simulink library "Lib_Sensors"  (R2014b)
settings: Solver=ode45  StartTime=0.0  StopTime=10.0  RelTol=1e-3
settings Model: Creator=Ehang  LastModifiedBy=Ehang

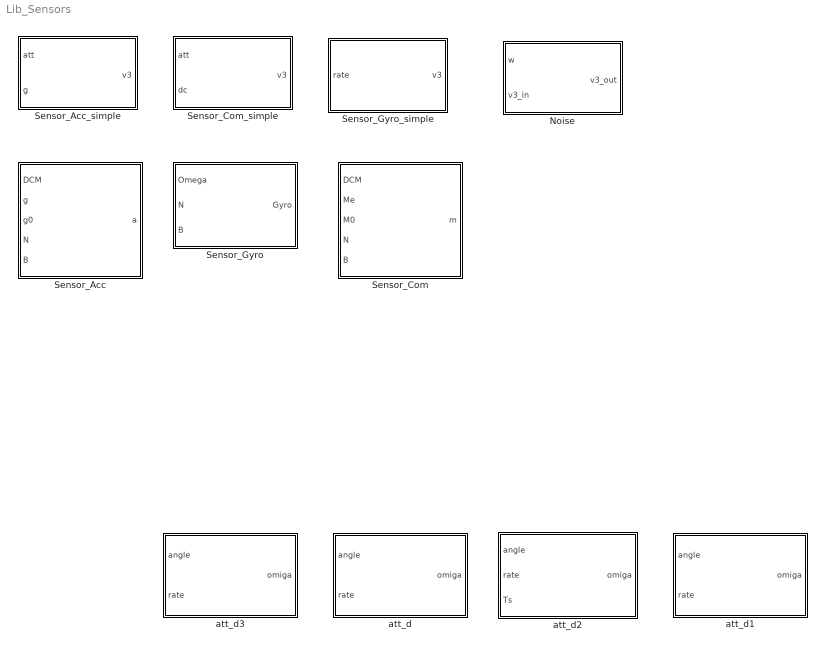
== system Lib_Sensors ==
  Noise : MATLAB Function  TreatAsAtomicUnit=on
  Sensor_Acc : Subsystem
  Sensor_Acc_simple : MATLAB Function  TreatAsAtomicUnit=on
  Sensor_Com : Subsystem
  Sensor_Com_simple : MATLAB Function  TreatAsAtomicUnit=on
  Sensor_Gyro : Subsystem
  Sensor_Gyro_simple : MATLAB Function  TreatAsAtomicUnit=on
  att_d : MATLAB Function  TreatAsAtomicUnit=on
  att_d1 : MATLAB Function  TreatAsAtomicUnit=on
  att_d2 : MATLAB Function  TreatAsAtomicUnit=on
  att_d3 : MATLAB Function  TreatAsAtomicUnit=on

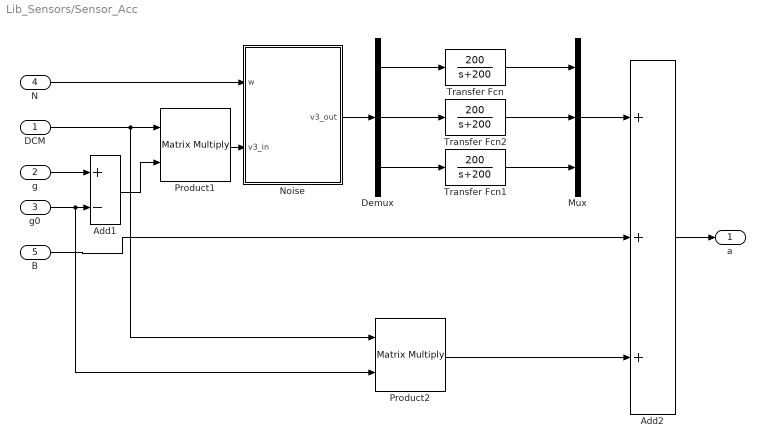
== system Lib_Sensors/Sensor_Acc ==
  DCM : Inport  PortDimensions=[3,3]
  g : Inport  Port=2
  g0 : Inport  Port=3
  N : Inport  Port=4  PortDimensions=[3,3]
  B : Inport  Port=5
  Add1 : Sum  Inputs=+-
  Add2 : Sum  Inputs=+++
  Demux : Demux  Outputs=3
  Mux : Mux  Inputs=3
  Noise : MATLAB Function  TreatAsAtomicUnit=on
  Product1 : Product  Multiplication=Matrix(*)
  Product2 : Product  Multiplication=Matrix(*)
  Transfer Fcn : TransferFcn  Numerator=[200]  Denominator=[1 200]
  Transfer Fcn1 : TransferFcn  Numerator=[200]  Denominator=[1 200]
  Transfer Fcn2 : TransferFcn  Numerator=[200]  Denominator=[1 200]
  a : Outport  PortDimensions=[3,1]
  wires:
  DCM/1 -> Product2/1, Product1/1
  Product1/1 -> Noise/2(v3_in)
  N/1 -> Noise/1(w)
  Noise/1(v3_out) -> Demux/1
  B/1 -> Add2/2
  Mux/1 -> Add2/1
  Transfer Fcn/1 -> Mux/1
  Demux/1 -> Transfer Fcn/1
  Transfer Fcn2/1 -> Mux/2
  Transfer Fcn1/1 -> Mux/3
  Demux/3 -> Transfer Fcn1/1
  Demux/2 -> Transfer Fcn2/1
  Add2/1 -> a/1
  g0/1 -> Product2/2, Add1/2
  g/1 -> Add1/1
  Add1/1 -> Product1/2
  Product2/1 -> Add2/3

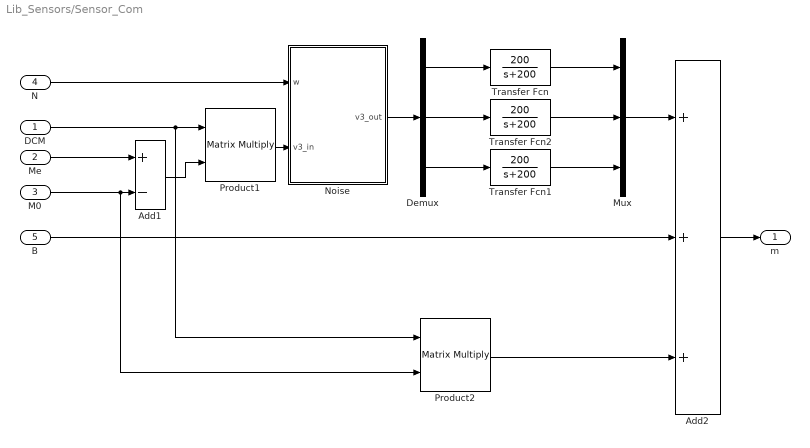
== system Lib_Sensors/Sensor_Com ==
  DCM : Inport  PortDimensions=[3,3]
  Me : Inport  Port=2
  M0 : Inport  Port=3
  N : Inport  Port=4  PortDimensions=[3,3]
  B : Inport  Port=5
  Add1 : Sum  Inputs=+-
  Add2 : Sum  Inputs=+++
  Demux : Demux  Outputs=3
  Mux : Mux  Inputs=3
  Noise : MATLAB Function  TreatAsAtomicUnit=on
  Product1 : Product  Multiplication=Matrix(*)
  Product2 : Product  Multiplication=Matrix(*)
  Transfer Fcn : TransferFcn  Numerator=[200]  Denominator=[1 200]
  Transfer Fcn1 : TransferFcn  Numerator=[200]  Denominator=[1 200]
  Transfer Fcn2 : TransferFcn  Numerator=[200]  Denominator=[1 200]
  m : Outport  PortDimensions=[3,1]
  wires:
  DCM/1 -> Product2/1, Product1/1
  Product1/1 -> Noise/2(v3_in)
  N/1 -> Noise/1(w)
  Noise/1(v3_out) -> Demux/1
  B/1 -> Add2/2
  Mux/1 -> Add2/1
  Transfer Fcn/1 -> Mux/1
  Demux/1 -> Transfer Fcn/1
  Transfer Fcn2/1 -> Mux/2
  Transfer Fcn1/1 -> Mux/3
  Demux/3 -> Transfer Fcn1/1
  Demux/2 -> Transfer Fcn2/1
  Add2/1 -> m/1
  M0/1 -> Product2/2, Add1/2
  Me/1 -> Add1/1
  Add1/1 -> Product1/2
  Product2/1 -> Add2/3

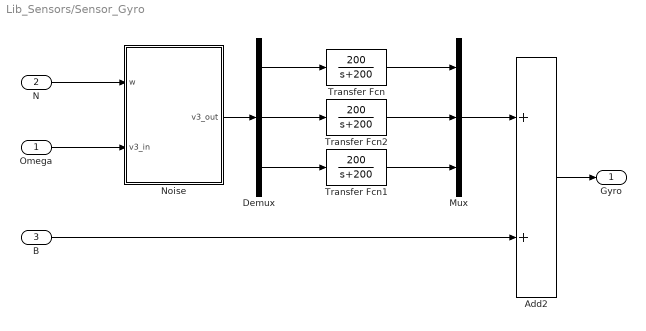
== system Lib_Sensors/Sensor_Gyro ==
  Omega : Inport
  N : Inport  Port=2  PortDimensions=[3,3]
  B : Inport  Port=3
  Add2 : Sum
  Demux : Demux  Outputs=3
  Mux : Mux  Inputs=3
  Noise : MATLAB Function  TreatAsAtomicUnit=on
  Transfer Fcn : TransferFcn  Numerator=[200]  Denominator=[1 200]
  Transfer Fcn1 : TransferFcn  Numerator=[200]  Denominator=[1 200]
  Transfer Fcn2 : TransferFcn  Numerator=[200]  Denominator=[1 200]
  Gyro : Outport  PortDimensions=[3,1]
  wires:
  Omega/1 -> Noise/2(v3_in)
  N/1 -> Noise/1(w)
  Noise/1(v3_out) -> Demux/1
  B/1 -> Add2/2
  Mux/1 -> Add2/1
  Transfer Fcn/1 -> Mux/1
  Demux/1 -> Transfer Fcn/1
  Transfer Fcn2/1 -> Mux/2
  Transfer Fcn1/1 -> Mux/3
  Demux/3 -> Transfer Fcn1/1
  Demux/2 -> Transfer Fcn2/1
  Add2/1 -> Gyro/1

== matlab function Lib_Sensors/Sensor_Acc/Noise ==
  data: w input size=[3,3]; v3_out output size=3; v3_in input size=3
function v3_out=Noise(w,v3_in)
v3_out=sqrt(w)*randn(3,1)+v3_in;

== matlab function Lib_Sensors/Sensor_Gyro/Noise ==
  data: w input size=[3,3]; v3_out output size=3; v3_in input size=3
function v3_out=Noise(w,v3_in)
v3_out=sqrt(w)*randn(3,1)+v3_in;

== matlab function Lib_Sensors/Sensor_Com/Noise ==
  data: w input size=[3,3]; v3_out output size=3; v3_in input size=3
function v3_out=Noise(w,v3_in)
v3_out=sqrt(w)*randn(3,1)+v3_in;

== matlab function Lib_Sensors/Sensor_Acc_simple ==
  data: att input size=3; v3 output size=3; g input
function v3=Acc_out(att,g)

roll=att(1);
pitch=att(2);
yaw=att(3);
cr=cos(roll);  sr=sin(roll);
cp=cos(pitch); sp=sin(pitch);
cy=cos(yaw);   sy=sin(yaw);
% syms cr sr cp sp cy sy
% RZ:Rotate Z axis
% RY:Rotate Y axis
% RX:Rotate X axis
% syms  RZ RY RX
%from earth to body
% RZ:Rotate Z axis
%右旋角度y为正
RZ = [  cy   sy   0;
       -sy   cy   0;
        0    0    1];

% RY:Rotate Y axis
%上仰角度P为正
RY = [  cp   0  -sp;
        0    1    0;
        sp   0   cp];

% RX:Rotate X axis
%右倾角度r为正
RX = [  1    0    0;
        0    cr  sr;
        0   -sr  cr];
%-----------------from_euler-----------------
% column : a b c
% row    : x y z
%                    a                 b      c
% x [            cp*cy,            cp*sy,   -sp]
% y [ cy*sp*sr - cr*sy, cr*cy + sp*sr*sy, cp*sr]
% z [ sr*sy + cr*cy*sp, cr*sp*sy - cy*sr, cp*cr]
% disp('Rotate Matix from earth fixed frame to body fixed frame;');
m= RX*RY*RZ;
% m= [            cp*cy,            cp*sy,   -sp;
%  cy*sp*sr - cr*sy, cr*cy + sp*sr*sy, cp*sr;
% sr*sy + cr*cy*sp, cr*sp*sy - cy*sr, cp*cr];
v3=g*dc;

== matlab function Lib_Sensors/att_d ==
  data: angle input size=3; rate input size=3; omiga output size=3
function omiga=att(angle,rate)
%% 用于在连续域解算欧拉角
%  yd  yaw的导数，pd  pitch的导数， rd roll的导数
% [p,q,r]'表示B系下飞行器绕自身旋转的角速度。
roll=angle(1);
pitch=angle(2);
yaw=angle(3);
p=rate(1);
q=rate(2);
r=rate(3);
%#codegen
cr=cos(roll);  sr=sin(roll);
cp=cos(pitch); sp=sin(pitch);
cy=cos(yaw);   sy=sin(yaw);
ab = [cp*cr     ,    -sr,      0;
      cp*sr     ,     cr,      0;
       -sp      ,      0,      1];
omiga=ab*[p,q,r]';

== matlab function Lib_Sensors/Sensor_Com_simple ==
  data: att input size=3; v3 output size=3; dc input
function v3=Com_out(att,dc)

roll=att(1);
pitch=att(2);
yaw=att(3);
cr=cos(roll);  sr=sin(roll);
cp=cos(pitch); sp=sin(pitch);
cy=cos(yaw);   sy=sin(yaw);
% syms cr sr cp sp cy sy
% RZ:Rotate Z axis
% RY:Rotate Y axis
% RX:Rotate X axis
% syms  RZ RY RX
%from earth to body
% RZ:Rotate Z axis
%右旋角度y为正
RZ = [  cy   sy   0;
       -sy   cy   0;
        0    0    1];

% RY:Rotate Y axis
%上仰角度P为正
RY = [  cp   0  -sp;
        0    1    0;
        sp   0   cp];

% RX:Rotate X axis
%右倾角度r为正
RX = [  1    0    0;
        0    cr  sr;
        0   -sr  cr];
%-----------------from_euler-----------------
% column : a b c
% row    : x y z
%                    a                 b      c
% x [            cp*cy,            cp*sy,   -sp]
% y [ cy*sp*sr - cr*sy, cr*cy + sp*sr*sy, cp*sr]
% z [ sr*sy + cr*cy*sp, cr*sp*sy - cy*sr, cp*cr]
% disp('Rotate Matix from earth fixed frame to body fixed frame;');
m= RX*RY*RZ;
% m= [            cp*cy,            cp*sy,   -sp;
%  cy*sp*sr - cr*sy, cr*cy + sp*sr*sy, cp*sr;
% sr*sy + cr*cy*sp, cr*sp*sy - cy*sr, cp*cr];
v3=m*dc;

== matlab function Lib_Sensors/att_d2 ==
  data: angle input; rate input; omiga output size=[3,1]; Ts input
function omiga=att(angle,rate,Ts)
%% 用于在离散域解算欧拉角
%  yd  yaw的导数，pd  pitch的导数， rd roll的导数
% [p,q,r]'表示B系下飞行器绕自身旋转的角速度。
roll=angle(1);
pitch=angle(2);
yaw=angle(3);
p=rate(1);
q=rate(2);
r=rate(3);
%#codegen
cr=cos(roll);  sr=sin(roll);
cp=cos(pitch); sp=sin(pitch);
cy=cos(yaw);   sy=sin(yaw);
ab = [cp*cr     ,    -sr,      0;
      cp*sr     ,     cr,      0;
       -sp      ,      0,      1];
omiga=Ts*ab*[p,q,r]';
omiga=angle+omiga;

== matlab function Lib_Sensors/Sensor_Gyro_simple ==
  data: rate input size=3; v3 output size=3
function v3=Gyro_out(rate)
v3=rate;

== matlab function Lib_Sensors/att_d1 ==
  data: angle input size=3; rate input size=3; omiga output size=3
function omiga=att(angle,rate)
%% 用于在连续域解算欧拉角
%  yd  yaw的导数，pd  pitch的导数， rd roll的导数
% [p,q,r]'表示B系下飞行器绕自身旋转的角速度。
roll=angle(1);
pitch=angle(2);
yaw=angle(3);
p=rate(1);
q=rate(2);
r=rate(3);
%#codegen
cr=cos(roll);  sr=sin(roll);
cp=cos(pitch); sp=sin(pitch);
cy=cos(yaw);   sy=sin(yaw);
ab = [cp*cr     ,    -sr,      0;
      cp*sr     ,     cr,      0;
       -sp      ,      0,      1];
omiga=inv(ab)*[p,q,r]';

== matlab function Lib_Sensors/att_d3 ==
  data: angle input size=3; rate input size=3; omiga output size=3
function omiga=att(angle,rate)
%% 用于在连续域解算欧拉角
%  yd  yaw的导数，pd  pitch的导数， rd roll的导数
% [p,q,r]'表示B系下飞行器绕自身旋转的角速度。
roll=angle(1);
pitch=angle(2);
yaw=angle(3);
p=rate(1);
q=rate(2);
r=rate(3);
%#codegen
cr=cos(roll);  sr=sin(roll);
cp=cos(pitch); sp=sin(pitch);
cy=cos(yaw);   sy=sin(yaw);
ab = [1     ,    sr*tan(pitch),      cr*tan(pitch);
      0     ,     cr,      -sr;
       0      ,      sr/cp,      cr/cp];
omiga=ab*[p,q,r]';

== matlab function Lib_Sensors/Noise ==
  data: w input size=[3,3]; v3_out output size=3; v3_in input size=3
function v3_out=Noise(w,v3_in)
v3_out=sqrt(w)*randn(3,1)+v3_in;
